simulink library "thrusterLib"  (R2015a)
settings: Solver=ode3  StartTime=0.0  StopTime=10.0  RelTol=1e-3
undefined symbols (not defined in the file): rho, thrusters
libraries: goto x10
settings Model: CovSFcnEnable=off  Creator=torstebo  LastModifiedBy=torstebo
settings DebuggingCC: UnderspecifiedInitializationDetection=Classic  MergeDetectMultiDrivingBlocksExec=none  SolverPrmCheckMsg=warning  StateNameClashWarn=warning

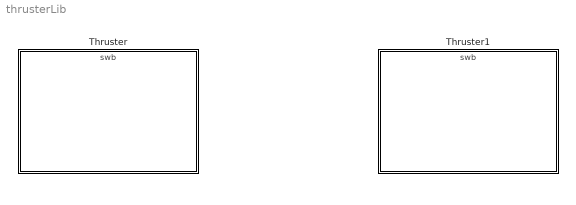
== system thrusterLib ==
  Thruster : Subsystem  Tag=Thruster  mask{thruster=thrusters(1), SwbId=1}
      mask prompts: thruster "Thruster data"; SwbId "Switchboard ID"
      mask Display:
      | image(imread('figs/thruster.jpg'))
      | color('black');
  Thruster1 : Subsystem  Tag=Thruster  mask{thruster=thrusters(1), SwbId=1}
      mask prompts: thruster "Thruster data"; SwbId "Switchboard ID"
      settings: AttributesFormatString=Simplefied %<thruster>
      mask Display:
      | image(imread('figs/thruster.jpg'))
      | color('black');

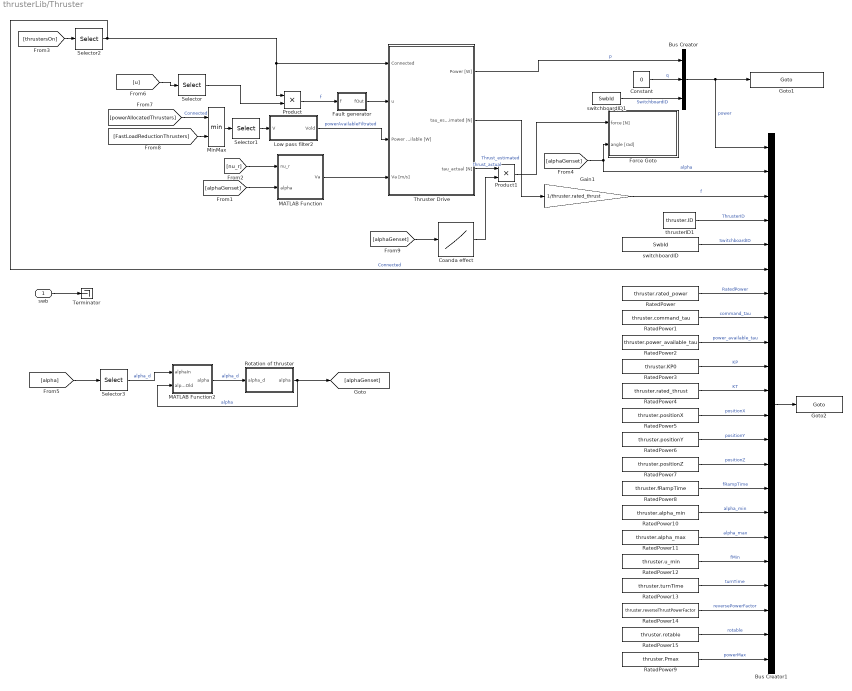
== system thrusterLib/Thruster ==
  swb : Inport
  Bus Creator : BusCreator  Inputs='p','q','SwitchboardID'  OutDataTypeStr=Bus: powerLoadsBus  NonVirtualBus=on
  Bus Creator1 : BusCreator  Inputs='power','alpha','f','ThrusterID','SwitchboardID','Connected','RatedPower','command_tau','power_available_tau','KP','KT','positionX','positionY','positionZ','fRampTime','alpha_min','alpha_max','fMin','turnTime','reversePowerFactor','rotable','powerMax'  OutDataTypeStr=Bus: ThrusterBus  NonVirtualBus=on
  Coanda effect : Lookup_n-D  NumberOfTableDimensions=1  BreakpointsForDimension1=[-2*pi,2*pi]  Table=[1,1]  RndMeth=Simplest  InputSameDT=on
  Constant : Constant  Value=0
  Fault generator : Subsystem
  Force Goto : Subsystem
  Gain1 : Gain  Gain=1/thruster.rated_thrust
  Goto1 : goto/Goto  GotoTag=sprintf('ThrusterPower%d',thruster.ID)
  Goto2 : goto/Goto  GotoTag=sprintf('Thruster%d',thruster.ID)
  Low pass filter2 : Subsystem
  MATLAB Function : MATLAB Function  TreatAsAtomicUnit=on
  MATLAB Function2 : MATLAB Function  TreatAsAtomicUnit=on
  MinMax : MinMax  Inputs=2
  Product : Product
  Product1 : Product
  RatedPower : Constant  Value=thruster.rated_power  OutDataTypeStr=double
  RatedPower1 : Constant  Value=thruster.command_tau  OutDataTypeStr=double
  RatedPower10 : Constant  Value=thruster.alpha_min  OutDataTypeStr=double
  RatedPower11 : Constant  Value=thruster.alpha_max  OutDataTypeStr=double
  RatedPower12 : Constant  Value=thruster.u_min  OutDataTypeStr=double
  RatedPower13 : Constant  Value=thruster.turnTime  OutDataTypeStr=double
  RatedPower14 : Constant  Value=thruster.reverseThrustPowerFactor  OutDataTypeStr=double
  RatedPower15 : Constant  Value=thruster.rotable  OutDataTypeStr=boolean
  RatedPower2 : Constant  Value=thruster.power_available_tau  OutDataTypeStr=double
  RatedPower3 : Constant  Value=thruster.KP0  OutDataTypeStr=double
  RatedPower4 : Constant  Value=thruster.rated_thrust  OutDataTypeStr=double
  RatedPower5 : Constant  Value=thruster.positionX  OutDataTypeStr=double
  RatedPower6 : Constant  Value=thruster.positionY  OutDataTypeStr=double
  RatedPower7 : Constant  Value=thruster.positionZ  OutDataTypeStr=double
  RatedPower8 : Constant  Value=thruster.fRampTime  OutDataTypeStr=double
  RatedPower9 : Constant  Value=thruster.Pmax  OutDataTypeStr=double
  Rotation of thruster : Subsystem
  Selector{,1..3} (4 alike) : Selector  Indices=thruster.ID
  Terminator : Terminator
  "Thruster Drive " : Subsystem
  switchboardID : Constant  Value=SwbId  OutDataTypeStr=uint8
  switchboardID1 : Constant  Value=SwbId  OutDataTypeStr=double
  thrusterID1 : Constant  Value=thruster.ID  OutDataTypeStr=uint8
  wires:
  Fault generator/1(fOut) -> "Thruster Drive "/2(u)
  Product/1 -> Fault generator/1(f)  "f"
  [alphaGenset] -> Coanda effect/1
  Coanda effect/1 -> Product1/2
  Product1/1 -> Force Goto/1(force [N])
  "Thruster Drive "/3(tau_actual [N]) -> Product1/1  "thrust_actual"
  MATLAB Function/1(Va) -> "Thruster Drive "/4(Va [m/s])
  [u] -> Selector/1
  [thrustersOn] -> Selector2/1
  [alphaGenset] -> Bus Creator1/2, Force Goto/2(angle [rad])  "alpha"
  Selector2/1 -> Bus Creator1/6, "Thruster Drive "/1(Connected), Product/1  "Connected"
  Selector/1 -> Product/2
  Selector1/1 -> Low pass filter2/1(V)
  Bus Creator/1 -> Goto1/1, Bus Creator1/1  "power"
  "Thruster Drive "/1(Power [W]) -> Bus Creator/1  "p"
  Constant/1 -> Bus Creator/2  "q"
  Low pass filter2/1(Vold) -> "Thruster Drive "/3(Power Available [W])  "powerAvailableFiltrated"
  MATLAB Function2/1(alpha) -> Rotation of thruster/1(alpha_d)  "alpha_d"
  [alpha] -> Selector3/1
  Rotation of thruster/1(alpha) -> [alphaGenset], MATLAB Function2/2(alphaOld)  "alpha"
  [alphaGenset] -> MATLAB Function/2(alpha)
  [nu_r] -> MATLAB Function/1(nu_r)
  Selector3/1 -> MATLAB Function2/1(alphaIn)  "alpha_d"
  MinMax/1 -> Selector1/1
  [FastLoadReductionThrusters] -> MinMax/2
  [powerAllocatedThrusters] -> MinMax/1  "Connected"
  switchboardID/1 -> Bus Creator1/5  "SwitchboardID"
  thrusterID1/1 -> Bus Creator1/4  "ThrusterID"
  RatedPower15/1 -> Bus Creator1/21  "rotable"
  RatedPower14/1 -> Bus Creator1/20  "reversePowerFactor"
  RatedPower13/1 -> Bus Creator1/19  "turnTime"
  RatedPower12/1 -> Bus Creator1/18  "fMin"
  RatedPower11/1 -> Bus Creator1/17  "alpha_max"
  RatedPower10/1 -> Bus Creator1/16  "alpha_min"
  RatedPower8/1 -> Bus Creator1/15  "fRampTime"
  RatedPower7/1 -> Bus Creator1/14  "positionZ"
  RatedPower6/1 -> Bus Creator1/13  "positionY"
  RatedPower5/1 -> Bus Creator1/12  "positionX"
  RatedPower4/1 -> Bus Creator1/11  "KT"
  RatedPower3/1 -> Bus Creator1/10  "KP"
  RatedPower2/1 -> Bus Creator1/9  "power_available_tau"
  RatedPower1/1 -> Bus Creator1/8  "command_tau"
  RatedPower/1 -> Bus Creator1/7  "RatedPower"
  Bus Creator1/1 -> Goto2/1
  swb/1 -> Terminator/1
  switchboardID1/1 -> Bus Creator/3  "SwitchboardID"
  RatedPower9/1 -> Bus Creator1/22  "powerMax"
  "Thruster Drive "/2(tau_estimated [N]) -> Gain1/1  "Thrust_estimated"
  Gain1/1 -> Bus Creator1/3  "f"

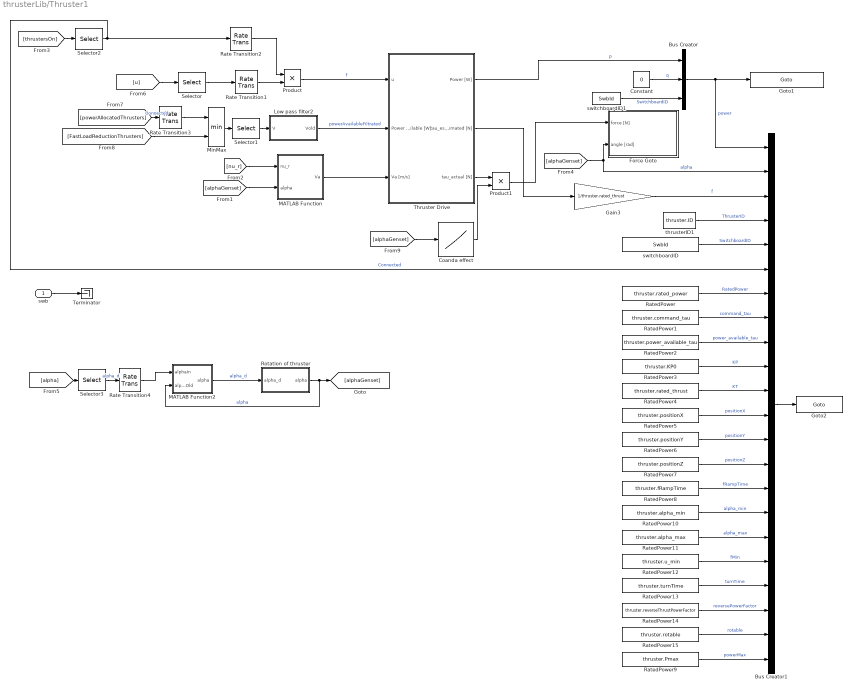
== system thrusterLib/Thruster1 ==
  swb : Inport
  Bus Creator : BusCreator  Inputs='p','q','SwitchboardID'  OutDataTypeStr=Bus: powerLoadsBus  NonVirtualBus=on
  Bus Creator1 : BusCreator  Inputs='power','alpha','f','ThrusterID','SwitchboardID','Connected','RatedPower','command_tau','power_available_tau','KP','KT','positionX','positionY','positionZ','fRampTime','alpha_min','alpha_max','fMin','turnTime','reversePowerFactor','rotable','powerMax'  OutDataTypeStr=Bus: ThrusterBus  NonVirtualBus=on
  Coanda effect : Lookup_n-D  NumberOfTableDimensions=1  BreakpointsForDimension1=[-2*pi,2*pi]  Table=[1,1]  RndMeth=Simplest  InputSameDT=on
  Constant : Constant  Value=0
  Force Goto : Subsystem
  Gain3 : Gain  Gain=1/thruster.rated_thrust  OutDataTypeStr=double
  Goto1 : goto/Goto  GotoTag=sprintf('ThrusterPower%d',thruster.ID)
  Goto2 : goto/Goto  GotoTag=sprintf('Thruster%d',thruster.ID)
  Low pass filter2 : Subsystem
  MATLAB Function : MATLAB Function  TreatAsAtomicUnit=on
  MATLAB Function2 : MATLAB Function  TreatAsAtomicUnit=on
  MinMax : MinMax  Inputs=2
  Product : Product
  Product1 : Product
  Rate Transition1 : RateTransition  Deterministic=off  X0=thruster.initial_thrust
  Rate Transition2 : RateTransition  X0=1
  Rate Transition3 : RateTransition  Deterministic=off  X0=thruster.rated_power
  Rate Transition4 : RateTransition  Deterministic=off  X0=thruster.alpha0
  RatedPower : Constant  Value=thruster.rated_power  OutDataTypeStr=double
  RatedPower1 : Constant  Value=thruster.command_tau  OutDataTypeStr=double
  RatedPower10 : Constant  Value=thruster.alpha_min  OutDataTypeStr=double
  RatedPower11 : Constant  Value=thruster.alpha_max  OutDataTypeStr=double
  RatedPower12 : Constant  Value=thruster.u_min  OutDataTypeStr=double
  RatedPower13 : Constant  Value=thruster.turnTime  OutDataTypeStr=double
  RatedPower14 : Constant  Value=thruster.reverseThrustPowerFactor  OutDataTypeStr=double
  RatedPower15 : Constant  Value=thruster.rotable  OutDataTypeStr=boolean
  RatedPower2 : Constant  Value=thruster.power_available_tau  OutDataTypeStr=double
  RatedPower3 : Constant  Value=thruster.KP0  OutDataTypeStr=double
  RatedPower4 : Constant  Value=thruster.rated_thrust  OutDataTypeStr=double
  RatedPower5 : Constant  Value=thruster.positionX  OutDataTypeStr=double
  RatedPower6 : Constant  Value=thruster.positionY  OutDataTypeStr=double
  RatedPower7 : Constant  Value=thruster.positionZ  OutDataTypeStr=double
  RatedPower8 : Constant  Value=thruster.fRampTime  OutDataTypeStr=double
  RatedPower9 : Constant  Value=thruster.Pmax  OutDataTypeStr=double
  Rotation of thruster : Subsystem
  Selector{,1..3} (4 alike) : Selector  Indices=thruster.ID
  Terminator : Terminator
  "Thruster Drive " : Subsystem
  switchboardID : Constant  Value=SwbId  OutDataTypeStr=uint8
  switchboardID1 : Constant  Value=SwbId  OutDataTypeStr=double
  thrusterID1 : Constant  Value=thruster.ID  OutDataTypeStr=uint8
  wires:
  Rate Transition3/1 -> MinMax/1
  Rate Transition2/1 -> Product/1
  Rate Transition1/1 -> Product/2
  Rate Transition4/1 -> MATLAB Function2/1(alphaIn)
  [alphaGenset] -> Coanda effect/1
  Coanda effect/1 -> Product1/2
  Product1/1 -> Force Goto/1(force [N])
  "Thruster Drive "/3(tau_actual [N]) -> Product1/1
  MATLAB Function/1(Va) -> "Thruster Drive "/3(Va [m/s])
  [u] -> Selector/1
  [thrustersOn] -> Selector2/1
  [alphaGenset] -> Bus Creator1/2, Force Goto/2(angle [rad])  "alpha"
  Selector2/1 -> Bus Creator1/6, Rate Transition2/1  "Connected"
  Selector/1 -> Rate Transition1/1
  Selector1/1 -> Low pass filter2/1(V)
  Gain3/1 -> Bus Creator1/3  "f"
  Bus Creator/1 -> Goto1/1, Bus Creator1/1  "power"
  "Thruster Drive "/1(Power [W]) -> Bus Creator/1  "p"
  Constant/1 -> Bus Creator/2  "q"
  Product/1 -> "Thruster Drive "/1(u)  "f"
  Low pass filter2/1(Vold) -> "Thruster Drive "/2(Power Available [W])  "powerAvailableFiltrated"
  MATLAB Function2/1(alpha) -> Rotation of thruster/1(alpha_d)  "alpha_d"
  [alpha] -> Selector3/1
  Rotation of thruster/1(alpha) -> [alphaGenset], MATLAB Function2/2(alphaOld)  "alpha"
  [alphaGenset] -> MATLAB Function/2(alpha)
  [nu_r] -> MATLAB Function/1(nu_r)
  Selector3/1 -> Rate Transition4/1  "alpha_d"
  MinMax/1 -> Selector1/1
  [FastLoadReductionThrusters] -> MinMax/2
  [powerAllocatedThrusters] -> Rate Transition3/1  "Connected"
  switchboardID/1 -> Bus Creator1/5  "SwitchboardID"
  thrusterID1/1 -> Bus Creator1/4  "ThrusterID"
  RatedPower15/1 -> Bus Creator1/21  "rotable"
  RatedPower14/1 -> Bus Creator1/20  "reversePowerFactor"
  RatedPower13/1 -> Bus Creator1/19  "turnTime"
  RatedPower12/1 -> Bus Creator1/18  "fMin"
  RatedPower11/1 -> Bus Creator1/17  "alpha_max"
  RatedPower10/1 -> Bus Creator1/16  "alpha_min"
  RatedPower8/1 -> Bus Creator1/15  "fRampTime"
  RatedPower7/1 -> Bus Creator1/14  "positionZ"
  RatedPower6/1 -> Bus Creator1/13  "positionY"
  RatedPower5/1 -> Bus Creator1/12  "positionX"
  RatedPower4/1 -> Bus Creator1/11  "KT"
  RatedPower3/1 -> Bus Creator1/10  "KP"
  RatedPower2/1 -> Bus Creator1/9  "power_available_tau"
  RatedPower1/1 -> Bus Creator1/8  "command_tau"
  RatedPower/1 -> Bus Creator1/7  "RatedPower"
  Bus Creator1/1 -> Goto2/1
  swb/1 -> Terminator/1
  switchboardID1/1 -> Bus Creator/3  "SwitchboardID"
  RatedPower9/1 -> Bus Creator1/22  "powerMax"
  "Thruster Drive "/2(tau_estimated [N]) -> Gain3/1

== system thrusterLib/Thruster/Fault generator ==
  f : Inport
  Constant : Constant  Value=thruster.fixThrust
  Step : Step  Time=thruster.fixThrustTime  SampleTime=0
  Switch : Switch  Criteria=u2 > Threshold
  fOut : Outport
  wires:
  f/1 -> Switch/3
  Step/1 -> Switch/2
  Constant/1 -> Switch/1
  Switch/1 -> fOut/1  "f"

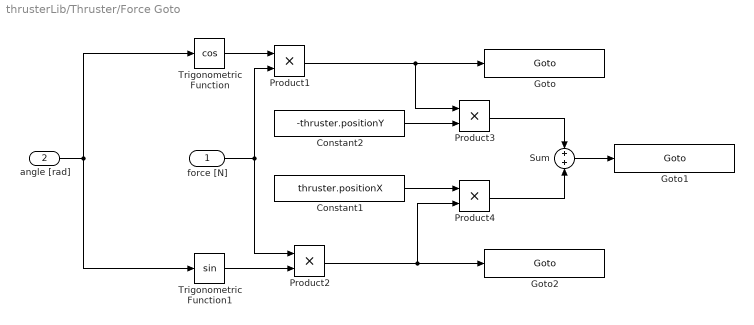
== system thrusterLib/Thruster/Force Goto ==
  force [N] : Inport
  angle [rad] : Inport  Port=2
  Constant1 : Constant  Value=thruster.positionX
  Constant2 : Constant  Value=-thruster.positionY
  Goto : goto/Goto  GotoTag=sprintf('ThrusterSurge%d',thruster.ID)
  Goto1 : goto/Goto  GotoTag=sprintf('ThrusterYaw%d',thruster.ID)
  Goto2 : goto/Goto  GotoTag=sprintf('ThrusterSway%d',thruster.ID)
  Product{1..4} (4 alike) : Product
  Sum : Sum
  Trigonometric Function : Trigonometry  Operator=cos
  Trigonometric Function1 : Trigonometry
  wires:
  Constant2/1 -> Product3/2
  Constant1/1 -> Product4/1
  Sum/1 -> Goto1/1
  Product3/1 -> Sum/1
  Product4/1 -> Sum/2
  Trigonometric Function1/1 -> Product2/2
  Product2/1 -> Goto2/1, Product4/2
  force [N]/1 -> Product1/2, Product2/1
  Trigonometric Function/1 -> Product1/1
  Product1/1 -> Goto/1, Product3/1
  angle [rad]/1 -> Trigonometric Function/1, Trigonometric Function1/1

== system thrusterLib/Thruster/Low pass filter2 ==
  V : Inport
  Gain : Gain  Gain=1/thruster.power_available_tau
  Integrator : Integrator  InitialCondition=thruster.rated_power
  Rate Limiter : RateLimiter  RisingSlewLimit=thruster.rated_power/thruster.power_available_positive_ramp_time  FallingSlewLimit=-inf  SampleTimeMode=inherited  InitialCondition=thruster.rated_power
  Sum : Sum  Inputs=|+-
  Vold : Outport
  wires:
  Gain/1 -> Integrator/1
  Sum/1 -> Gain/1
  Integrator/1 -> Sum/2, Rate Limiter/1
  V/1 -> Sum/1
  Rate Limiter/1 -> Vold/1

== system thrusterLib/Thruster/Rotation of thruster ==
  alpha_d : Inport
  Gain : Gain  Gain=1/thruster.Talpha
  Integrator : Integrator  InitialCondition=thruster.alpha0
  Rate Limiter : RateLimiter  RisingSlewLimit=2*pi/thruster.turnTime  FallingSlewLimit=-2*pi/thruster.turnTime  SampleTimeMode=inherited  InitialCondition=thruster.alpha0
  Saturation : Saturate  UpperLimit=thruster.alpha_max  LowerLimit=thruster.alpha_min
  Sum : Sum  Inputs=|+-
  alpha : Outport
  wires:
  Saturation/1 -> Rate Limiter/1
  Rate Limiter/1 -> Sum/1
  Gain/1 -> Integrator/1
  Sum/1 -> Gain/1
  Integrator/1 -> alpha/1, Sum/2
  alpha_d/1 -> Saturation/1

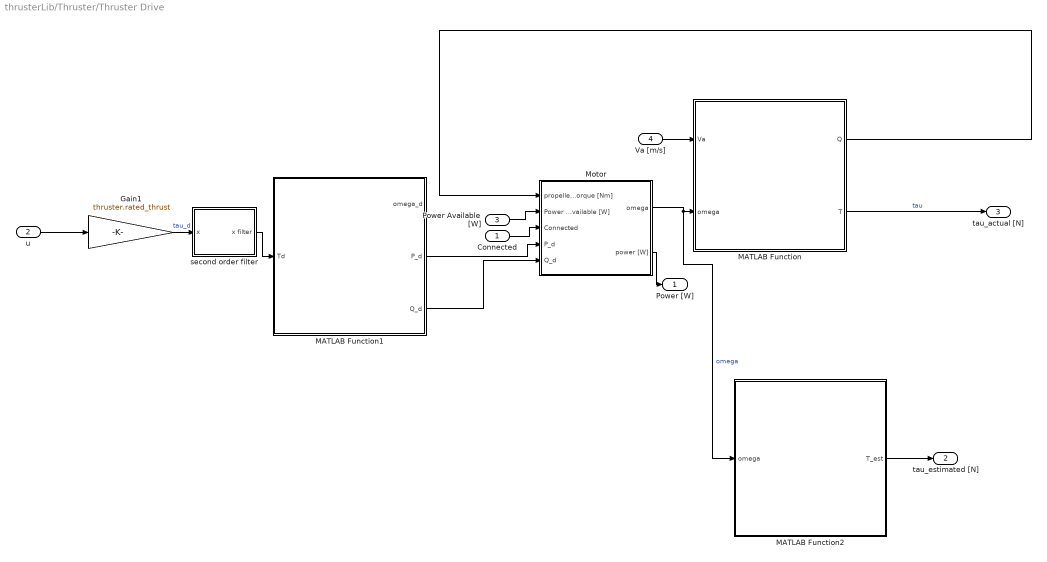
== system thrusterLib/Thruster/Thruster Drive  ==
  Connected : Inport
  u : Inport  Port=2
  Power Available [W] : Inport  Port=3
  Va [m/s] : Inport  Port=4
  Gain1 : Gain  Gain=thruster.rated_thrust
  MATLAB Function : MATLAB Function  TreatAsAtomicUnit=on
  MATLAB Function1 : MATLAB Function  TreatAsAtomicUnit=on
  MATLAB Function2 : MATLAB Function  TreatAsAtomicUnit=on
  Motor : Subsystem
  second order filter : Subsystem  mask{w0=2*pi/thruster.omega_ref_tau, xi=1, x_init=thruster.initial_thrust, dx_init=0}
      mask prompts: w0 "Frequency"; xi "Damping"; x_init "Initial condition"; dx_init "Initial time derivative"
  Power [W] : Outport
  tau_estimated [N] : Outport  Port=2
  tau_actual [N] : Outport  Port=3
  wires:
  MATLAB Function1/2(P_d) -> Motor/4(P_d)
  MATLAB Function1/3(Q_d) -> Motor/5(Q_d)
  second order filter/1(x filter) -> MATLAB Function1/1(Td)
  Va [m/s]/1 -> MATLAB Function/1(Va)
  MATLAB Function/1(Q) -> Motor/1(propeller torque [Nm])
  Motor/1(omega) -> MATLAB Function2/1(omega), MATLAB Function/2(omega)  "omega"
  u/1 -> Gain1/1
  Power Available [W]/1 -> Motor/2(Power Available [W])
  Gain1/1 -> second order filter/1(x)  "tau_d"
  MATLAB Function/2(T) -> tau_actual [N]/1  "tau"
  Motor/2(power [W]) -> Power [W]/1
  Connected/1 -> Motor/3(Connected)
  MATLAB Function2/1(T_est) -> tau_estimated [N]/1

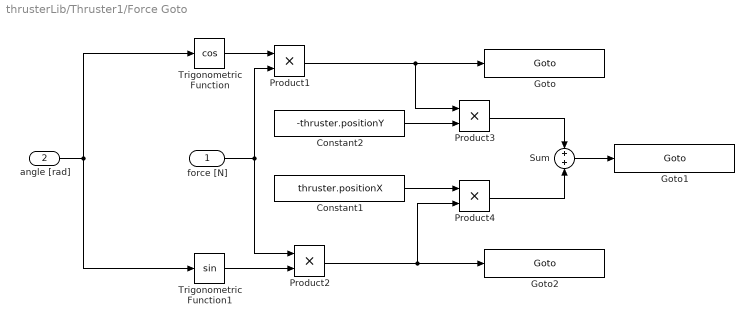
== system thrusterLib/Thruster1/Force Goto ==
  force [N] : Inport
  angle [rad] : Inport  Port=2
  Constant1 : Constant  Value=thruster.positionX
  Constant2 : Constant  Value=-thruster.positionY
  Goto : goto/Goto  GotoTag=sprintf('ThrusterSurge%d',thruster.ID)
  Goto1 : goto/Goto  GotoTag=sprintf('ThrusterYaw%d',thruster.ID)
  Goto2 : goto/Goto  GotoTag=sprintf('ThrusterSway%d',thruster.ID)
  Product{1..4} (4 alike) : Product
  Sum : Sum
  Trigonometric Function : Trigonometry  Operator=cos
  Trigonometric Function1 : Trigonometry
  wires:
  Constant2/1 -> Product3/2
  Constant1/1 -> Product4/1
  Sum/1 -> Goto1/1
  Product3/1 -> Sum/1
  Product4/1 -> Sum/2
  Trigonometric Function1/1 -> Product2/2
  Product2/1 -> Goto2/1, Product4/2
  force [N]/1 -> Product1/2, Product2/1
  Trigonometric Function/1 -> Product1/1
  Product1/1 -> Goto/1, Product3/1
  angle [rad]/1 -> Trigonometric Function/1, Trigonometric Function1/1

== system thrusterLib/Thruster1/Low pass filter2 ==
  V : Inport
  Gain : Gain  Gain=1/thruster.power_available_tau
  Integrator : Integrator  InitialCondition=thruster.rated_power
  Rate Limiter : RateLimiter  RisingSlewLimit=thruster.rated_power/thruster.power_available_positive_ramp_time  FallingSlewLimit=-inf  SampleTimeMode=inherited  InitialCondition=thruster.rated_power
  Sum : Sum  Inputs=|+-
  Vold : Outport
  wires:
  Gain/1 -> Integrator/1
  Sum/1 -> Gain/1
  Integrator/1 -> Sum/2, Rate Limiter/1
  V/1 -> Sum/1
  Rate Limiter/1 -> Vold/1

== system thrusterLib/Thruster1/Rotation of thruster ==
  alpha_d : Inport
  Gain : Gain  Gain=1/thruster.Talpha
  Integrator : Integrator  InitialCondition=thruster.alpha0
  Rate Limiter : RateLimiter  RisingSlewLimit=2*pi/thruster.turnTime  FallingSlewLimit=-2*pi/thruster.turnTime  SampleTimeMode=inherited  InitialCondition=thruster.alpha0
  Saturation : Saturate  UpperLimit=thruster.alpha_max  LowerLimit=thruster.alpha_min
  Sum : Sum  Inputs=|+-
  alpha : Outport
  wires:
  Saturation/1 -> Rate Limiter/1
  Rate Limiter/1 -> Sum/1
  Gain/1 -> Integrator/1
  Sum/1 -> Gain/1
  Integrator/1 -> alpha/1, Sum/2
  alpha_d/1 -> Saturation/1

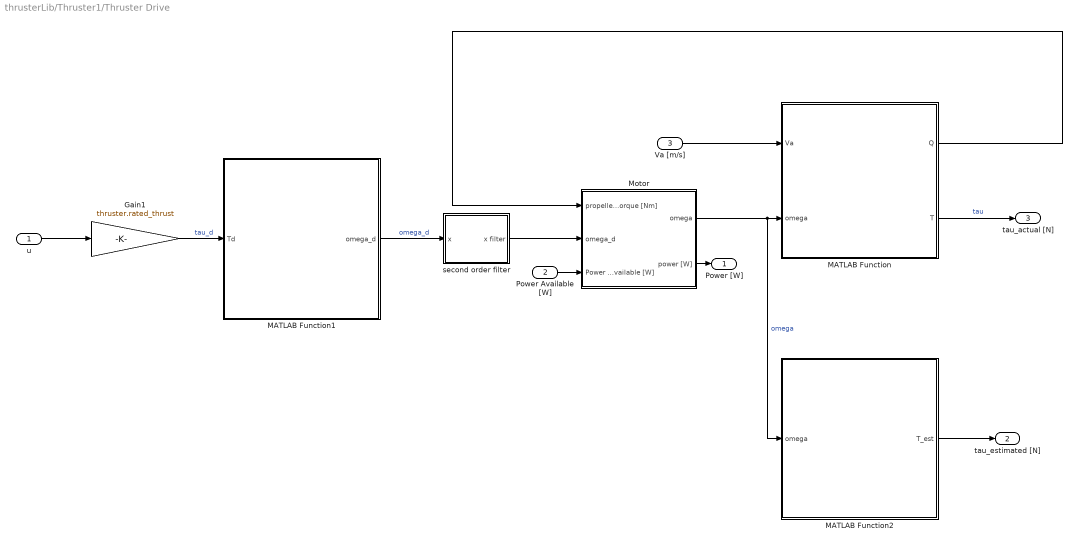
== system thrusterLib/Thruster1/Thruster Drive  ==
  u : Inport
  Power Available [W] : Inport  Port=2
  Va [m/s] : Inport  Port=3
  Gain1 : Gain  Gain=thruster.rated_thrust
  MATLAB Function : MATLAB Function  TreatAsAtomicUnit=on
  MATLAB Function1 : MATLAB Function  TreatAsAtomicUnit=on
  MATLAB Function2 : MATLAB Function  TreatAsAtomicUnit=on
  Motor : Subsystem
  second order filter : Subsystem  mask{w0=2*pi/thruster.omega_ref_tau, xi=1, x_init=thruster.motor.omega0/thruster.k_g, dx_init=0}
      mask prompts: w0 "Frequency"; xi "Damping"; x_init "Initial condition"; dx_init "Initial time derivative"
  Power [W] : Outport
  tau_estimated [N] : Outport  Port=2
  tau_actual [N] : Outport  Port=3
  wires:
  Va [m/s]/1 -> MATLAB Function/1(Va)
  MATLAB Function/1(Q) -> Motor/1(propeller torque [Nm])
  MATLAB Function1/1(omega_d) -> second order filter/1(x)  "omega_d"
  u/1 -> Gain1/1
  Power Available [W]/1 -> Motor/3(Power Available [W])
  Gain1/1 -> MATLAB Function1/1(Td)  "tau_d"
  MATLAB Function/2(T) -> tau_actual [N]/1  "tau"
  Motor/2(power [W]) -> Power [W]/1
  second order filter/1(x filter) -> Motor/2(omega_d)
  MATLAB Function2/1(T_est) -> tau_estimated [N]/1
  Motor/1(omega) -> MATLAB Function2/1(omega), MATLAB Function/2(omega)  "omega"

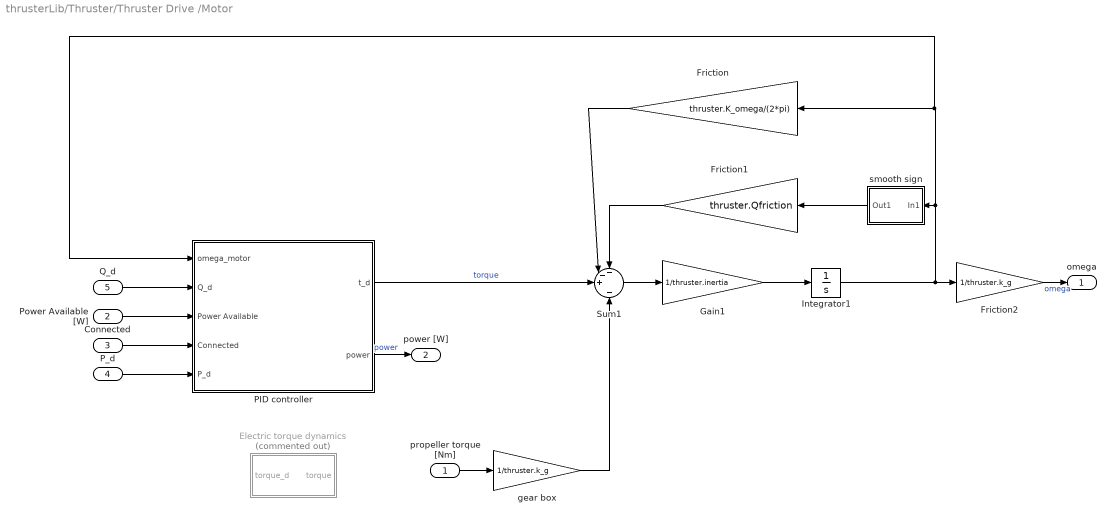
== system thrusterLib/Thruster/Thruster Drive /Motor ==
  propeller torque [Nm] : Inport
  Power Available [W] : Inport  Port=2
  Connected : Inport  Port=3
  P_d : Inport  Port=4
  Q_d : Inport  Port=5
  Electric torque dynamics : Subsystem  Commented=on
  Friction : Gain  Gain=thruster.K_omega/(2*pi)
  Friction1 : Gain  Gain=thruster.Qfriction
  Friction2 : Gain  Gain=1/thruster.k_g
  Gain1 : Gain  Gain=1/thruster.inertia
  Integrator1 : Integrator  InitialCondition=thruster.motor.omega0
  PID controller : Subsystem
  Sum1 : Sum  Inputs=--+|-
  gear box : Gain  Gain=1/thruster.k_g
  smooth sign : Subsystem
  omega : Outport
  power [W] : Outport  Port=2
  wires:
  P_d/1 -> PID controller/5(P_d)
  Q_d/1 -> PID controller/2(Q_d)
  Power Available [W]/1 -> PID controller/3(Power Available)
  propeller torque [Nm]/1 -> gear box/1
  Friction2/1 -> omega/1  "omega"
  Friction1/1 -> Sum1/1
  smooth sign/1(Out1) -> Friction1/1
  PID controller/2(power) -> power [W]/1  "power"
  PID controller/1(t_d) -> Sum1/3  "torque"
  Friction/1 -> Sum1/2
  gear box/1 -> Sum1/4
  Gain1/1 -> Integrator1/1
  Sum1/1 -> Gain1/1
  Integrator1/1 -> Friction2/1, smooth sign/1(In1), Friction/1, PID controller/1(omega_motor)
  Connected/1 -> PID controller/4(Connected)

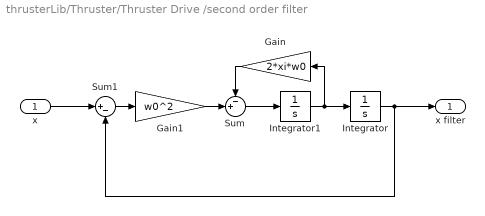
== system thrusterLib/Thruster/Thruster Drive /second order filter ==
  x : Inport
  Gain : Gain  Gain=2*xi*w0
  Gain1 : Gain  Gain=w0^2
  Integrator : Integrator  InitialCondition=x_init
  Integrator1 : Integrator  InitialCondition=dx_init
  Sum : Sum  Inputs=-+|
  Sum1 : Sum  Inputs=|+-
  x filter : Outport
  wires:
  Sum1/1 -> Gain1/1
  Gain1/1 -> Sum/2
  Integrator/1 -> Sum1/2, x filter/1
  Sum/1 -> Integrator1/1
  x/1 -> Sum1/1
  Integrator1/1 -> Integrator/1, Gain/1
  Gain/1 -> Sum/1

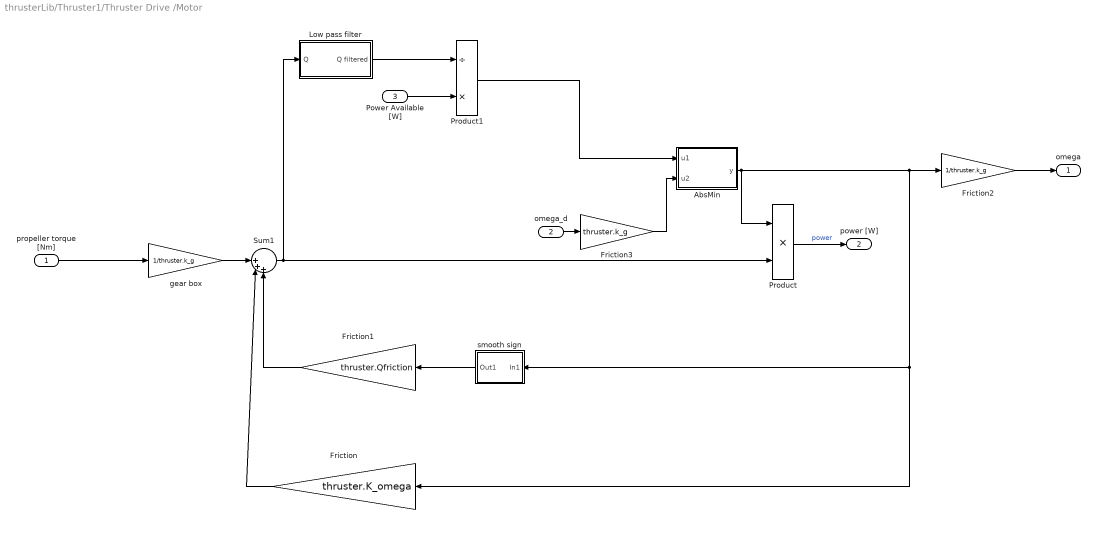
== system thrusterLib/Thruster1/Thruster Drive /Motor ==
  propeller torque [Nm] : Inport
  omega_d : Inport  Port=2
  Power Available [W] : Inport  Port=3
  AbsMin : MATLAB Function  TreatAsAtomicUnit=on
  Friction : Gain  Gain=thruster.K_omega
  Friction1 : Gain  Gain=thruster.Qfriction
  Friction2 : Gain  Gain=1/thruster.k_g
  Friction3 : Gain  Gain=thruster.k_g
  Low pass filter : Subsystem
  Product : Product
  Product1 : Product  Inputs=/*
  Sum1 : Sum  Inputs=||+++
  gear box : Gain  Gain=1/thruster.k_g
  smooth sign : Subsystem
  omega : Outport
  power [W] : Outport  Port=2
  wires:
  Friction3/1 -> AbsMin/2(u2)
  AbsMin/1(y) -> Product/1, Friction2/1, smooth sign/1(In1), Friction/1
  propeller torque [Nm]/1 -> gear box/1
  smooth sign/1(Out1) -> Friction1/1
  Product/1 -> power [W]/1  "power"
  gear box/1 -> Sum1/1
  Sum1/1 -> Low pass filter/1(Q), Product/2
  Friction2/1 -> omega/1
  Power Available [W]/1 -> Product1/2
  Product1/1 -> AbsMin/1(u1)
  omega_d/1 -> Friction3/1
  Low pass filter/1(Q filtered) -> Product1/1
  Friction/1 -> Sum1/2
  Friction1/1 -> Sum1/3

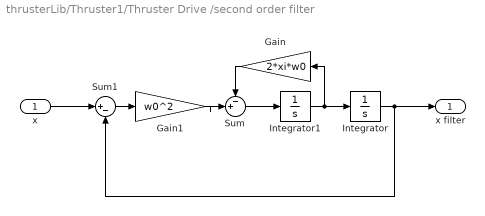
== system thrusterLib/Thruster1/Thruster Drive /second order filter ==
  x : Inport
  Gain : Gain  Gain=2*xi*w0
  Gain1 : Gain  Gain=w0^2
  Integrator : Integrator  InitialCondition=x_init
  Integrator1 : Integrator  InitialCondition=dx_init
  Sum : Sum  Inputs=-+|
  Sum1 : Sum  Inputs=|+-
  x filter : Outport
  wires:
  Sum1/1 -> Gain1/1
  Gain1/1 -> Sum/2
  Integrator/1 -> Sum1/2, x filter/1
  Sum/1 -> Integrator1/1
  x/1 -> Sum1/1
  Integrator1/1 -> Integrator/1, Gain/1
  Gain/1 -> Sum/1

== system thrusterLib/Thruster/Thruster Drive /Motor/Electric torque dynamics ==
  torque_d : Inport
  Gain : Gain  Gain=1/thruster.motor.T
  Integrator : Integrator  InitialCondition=thruster.motor.torque0
  Sum : Sum  Inputs=|+-
  torque : Outport
  wires:
  Integrator/1 -> Sum/2, torque/1
  torque_d/1 -> Sum/1
  Sum/1 -> Gain/1
  Gain/1 -> Integrator/1

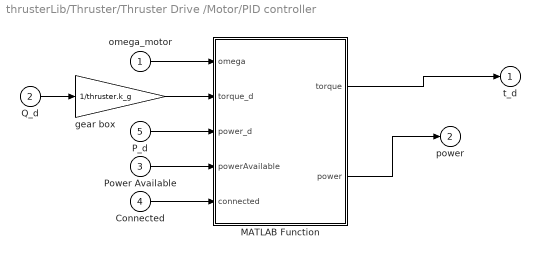
== system thrusterLib/Thruster/Thruster Drive /Motor/PID controller ==
  omega_motor : Inport  PortDimensions=1
  Q_d : Inport  Port=2  PortDimensions=1
  Power Available : Inport  Port=3  PortDimensions=1
  Connected : Inport  Port=4  PortDimensions=1
  P_d : Inport  Port=5  PortDimensions=1
  MATLAB Function : MATLAB Function  TreatAsAtomicUnit=on
  gear box : Gain  Gain=1/thruster.k_g
  t_d : Outport  PortDimensions=1  InitialOutput=0
  power : Outport  Port=2  PortDimensions=1  InitialOutput=0
  wires:
  gear box/1 -> MATLAB Function/2(torque_d)
  P_d/1 -> MATLAB Function/3(power_d)
  MATLAB Function/2(power) -> power/1
  Power Available/1 -> MATLAB Function/4(powerAvailable)
  Connected/1 -> MATLAB Function/5(connected)
  omega_motor/1 -> MATLAB Function/1(omega)
  MATLAB Function/1(torque) -> t_d/1
  Q_d/1 -> gear box/1

== system thrusterLib/Thruster/Thruster Drive /Motor/smooth sign ==
  In1 : Inport
  Friction1 : Gain  Gain=100
  Trigonometric Function : Trigonometry  Operator=tanh
  Out1 : Outport
  wires:
  In1/1 -> Friction1/1
  Trigonometric Function/1 -> Out1/1
  Friction1/1 -> Trigonometric Function/1

== system thrusterLib/Thruster1/Thruster Drive /Motor/Low pass filter ==
  Q : Inport
  Gain : Gain  Gain=1/.5
  Integrator : Integrator
  Sum : Sum  Inputs=|+-
  Q filtered : Outport
  wires:
  Gain/1 -> Integrator/1
  Sum/1 -> Gain/1
  Q/1 -> Sum/1
  Integrator/1 -> Sum/2, Q filtered/1

== system thrusterLib/Thruster1/Thruster Drive /Motor/smooth sign ==
  In1 : Inport
  Friction1 : Gain  Gain=100
  Trigonometric Function : Trigonometry  Operator=tanh
  Out1 : Outport
  wires:
  In1/1 -> Friction1/1
  Trigonometric Function/1 -> Out1/1
  Friction1/1 -> Trigonometric Function/1

== matlab function thrusterLib/Thruster1/MATLAB Function2 ==
  data: alphaIn input; alpha output; alphaOld input
function alpha = remap(alphaIn,alphaOld)
%#codegen

dalpha = mod(alphaIn-alphaOld,2*pi);
% Map dalpha to (-pi pi]
dalpha = (dalpha > pi).*(-2*pi)+dalpha;
alpha = alphaOld + dalpha;

== matlab function thrusterLib/Thruster/MATLAB Function ==
  data: nu_r input; Va output; thruster parameter; alpha input
function Va = fcn(nu_r,thruster,alpha)
%#codegen
r = [thruster.positionX;thruster.positionY];
v = nu_r(1:2)+nu_r(6)*r;
Va = v.'*[cos(alpha);sin(alpha)];

== matlab function thrusterLib/Thruster1/Thruster Drive /MATLAB Function2 ==
  data: omega input; T_est output; thruster parameter; rho parameter
function T_est  = propeller(omega,thruster,rho)
%#codegen
T_est = estimatedThrusterForce(omega,thruster,rho);

== matlab function thrusterLib/Thruster/MATLAB Function2 ==
  data: alphaIn input; alpha output; alphaOld input
function alpha = remap(alphaIn,alphaOld)
%#codegen

dalpha = mod(alphaIn-alphaOld,2*pi);
% Map dalpha to (-pi pi]
dalpha = (dalpha > pi).*(-2*pi)+dalpha;
alpha = alphaOld + dalpha;

== matlab function thrusterLib/Thruster1/Thruster Drive /Motor/AbsMin ==
  data: u1 input; y output; u2 input
function y = absMin(u1,u2)
%#codegen
if (isnan(u1) || isinf(u1))
    y=u2;
elseif (isnan(u2) || isinf(u2))   
    y=u1 ;
elseif(abs(u1)>abs(u2))
    y=u2;
else
    y=u1;
end

== matlab function thrusterLib/Thruster1/MATLAB Function ==
  data: nu_r input; Va output; thruster parameter; alpha input
function Va = fcn(nu_r,thruster,alpha)
%#codegen
r = [thruster.positionX;thruster.positionY];
v = nu_r(1:2)+nu_r(3)*r;
Va = v.'*[cos(alpha);sin(alpha)];

== matlab function thrusterLib/Thruster1/Thruster Drive /MATLAB Function ==
  data: Q output; Va input; omega input; T output; thruster parameter; rho parameter
function [Q,T] = propeller(Va,omega,thruster,rho)
%#codegen
beta = atan2(Va,0.7*pi*omega*thruster.radius);
Ct = 0;
Cq = 0;
for i = 1:length(thruster.AT)
    Ct = Ct + thruster.AT(i)*cos(beta*(i-1))+thruster.BT(i)*sin(beta*(i-1));
    Cq = Cq + thruster.AQ(i)*cos(beta*(i-1))+thruster.BQ(i)*sin(beta*(i-1));
end
V07_2 = Va^2+(0.7*omega*thruster.radius)^2;
T = Ct*.5*rho*V07_2*pi*thruster.radius^2;
Q = Cq*.5*rho*V07_2*pi*2*thruster.radius^3;

== matlab function thrusterLib/Thruster1/Thruster Drive /MATLAB Function1 ==
  data: Td input; omega_d output; thruster parameter; rho parameter
function omega_d  = propeller(Td,thruster,rho)
%#codegen
omega_d = findDesiredPropellerSpeed(Td,thruster,rho);

== matlab function thrusterLib/Thruster/Thruster Drive /MATLAB Function ==
  data: Q output; Va input; omega input; T output; thruster parameter; rho parameter
function [Q,T] = propeller(Va,omega,thruster,rho)
%#codegen
beta = atan2(Va,0.7*pi*omega*thruster.radius);
Ct = 0;
Cq = 0;
for i = 1:length(thruster.AT)
    Ct = Ct + thruster.AT(i)*cos(beta*(i-1))+thruster.BT(i)*sin(beta*(i-1));
    Cq = Cq + thruster.AQ(i)*cos(beta*(i-1))+thruster.BQ(i)*sin(beta*(i-1));
end
V07_2 = Va^2+(0.7*omega*thruster.radius)^2;
T = Ct*.5*rho*V07_2*pi*thruster.radius^2;
Q = Cq*.5*rho*V07_2*pi*2*thruster.radius^3;

== matlab function thrusterLib/Thruster/Thruster Drive /MATLAB Function1 ==
  data: Td input; omega_d output; thruster parameter; rho parameter; P_d output; Q_d output
function [omega_d, P_d, Q_d]  = propeller(Td,thruster,rho)
%#codegen
[omega_d, P_d, Q_d] = findDesiredPropellerSpeed(Td,thruster,rho);

== matlab function thrusterLib/Thruster/Thruster Drive /MATLAB Function2 ==
  data: omega input; T_est output; thruster parameter; rho parameter
function T_est  = propeller(omega,thruster,rho)
%#codegen
T_est = estimatedThrusterForce(omega,thruster,rho);

== matlab function thrusterLib/Thruster/Thruster Drive /Motor/PID controller/MATLAB Function ==
  data: omega input; torque_d input; power_d input; torque output; thruster parameter; power output; powerAvailable input; connected input
function [torque, power] = saturation(omega,torque_d, power_d,thruster,powerAvailable, connected)
%#codegen
if (powerAvailable <= .1 || ~connected)
    power = 0;
    torque = 0;
    return
end

k = 4;
p = 1;
r = 2;
alpha = exp(-k*abs(p*omega/(2*pi))^r);
torque_d = power_d/omega*(1-alpha)+alpha*torque_d;

% check for inverse power
if (omega*torque_d<-thruster.motor.maxReversePower)
    torque = -thruster.motor.maxReversePower/omega;
    power = -thruster.motor.maxReversePower;
    return
end

% check maximum torque
torque_d = sign(torque_d)*min(thruster.Qmax,abs(torque_d));

% check maximum power (has checked for inverse power)
pMax = min(thruster.Pmax,powerAvailable);
if (omega*torque_d>pMax)
    torque_d = torque_d*(pMax/(omega*torque_d));
end

torque = torque_d;
power = torque*omega;
